simulink library "controller_lib"  (R2022b)
settings: Solver=VariableStepAuto  StartTime=0.0  StopTime=10.0  RelTol=1e-3
libraries: battery_monitor_lib x1, driver_interface_lib x1, governor_lib x1, motor_interface_lib x1, vehicle_dynamics_lib x1
settings Model: Creator=dr_pa  LastModifiedBy=dr_pa

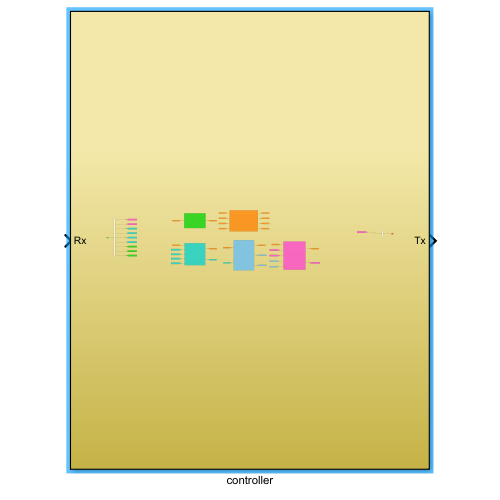
[thumbnail: Simulink's stored preview of the top-level diagram]
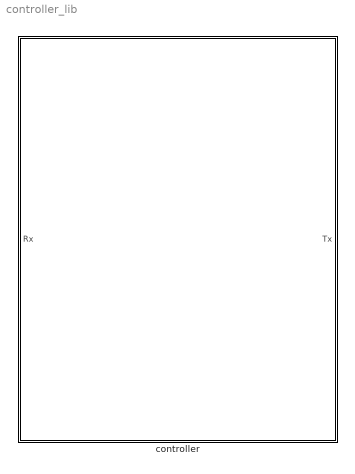
== system controller_lib ==
  controller : Subsystem

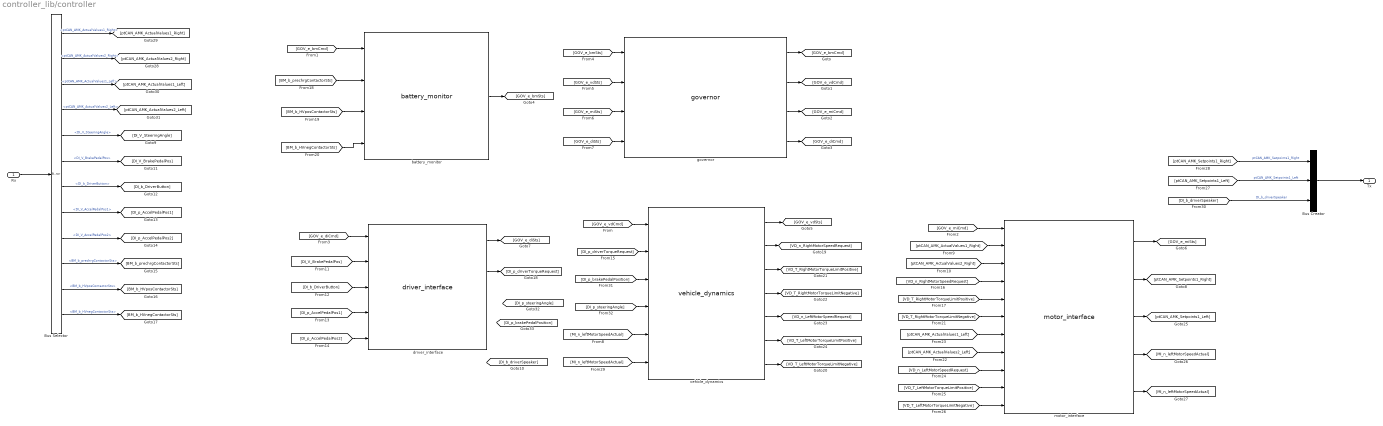
== system controller_lib/controller ==
  Rx : Inport
  Bus Creator : BusCreator  Inputs=3
  Bus Selector : BusSelector  OutputSignals=ptCAN_AMK_ActualValues1_Right,ptCAN_AMK_ActualValues2_Right,ptCAN_AMK_ActualValues1_Left,ptCAN_AMK_ActualValues2_Left,DI_V_SteeringAngle,DI_V_BrakePedalPos,DI_b_DriverButton,DI_V_AccelPedalPos1,DI_V_AccelPedalPos2,BM_b_prechrgContactorSts,BM_b_HVposContactorSts,BM_b_HVnegContactorSts
  battery_monitor : battery_monitor_lib/battery_monitor  SystemSampleTime=-1  VariantActivationTime=update diagram  Latency=0  AutoFrameSizeCalculation=off
  driver_interface : driver_interface_lib/driver_interface  SystemSampleTime=-1  VariantActivationTime=update diagram  Latency=0  AutoFrameSizeCalculation=off
  governor : governor_lib/governor  SystemSampleTime=-1  VariantActivationTime=update diagram  Latency=0  AutoFrameSizeCalculation=off
  motor_interface : motor_interface_lib/motor_interface  SystemSampleTime=-1  VariantActivationTime=update diagram  Latency=0  AutoFrameSizeCalculation=off
  vehicle_dynamics : vehicle_dynamics_lib/vehicle_dynamics  SystemSampleTime=-1  VariantActivationTime=update diagram  Latency=0  AutoFrameSizeCalculation=off
  Tx : Outport
  wires:
  governor/1 -> [GOV_e_bmCmd]
  [GOV_e_vdCmd] -> vehicle_dynamics/1
  governor/2 -> [GOV_e_vdCmd]
  governor/3 -> [GOV_e_miCmd]
  [GOV_e_miCmd] -> motor_interface/1
  governor/4 -> [GOV_e_diCmd]
  [GOV_e_diCmd] -> driver_interface/1
  battery_monitor/1 -> [GOV_e_bmSts]
  [GOV_e_bmSts] -> governor/1
  vehicle_dynamics/1 -> [GOV_e_vdSts]
  [GOV_e_vdSts] -> governor/2
  motor_interface/1 -> [GOV_e_miSts]
  [GOV_e_miSts] -> governor/3
  [GOV_e_diSts] -> governor/4
  driver_interface/1 -> [GOV_e_diSts]
  Bus Creator/1 -> Tx/1
  [ptCAN_AMK_Setpoints1_Right] -> Bus Creator/1  "ptCAN_AMK_Setpoints1_Right"
  motor_interface/2 -> [ptCAN_AMK_Setpoints1_Right]
  [ptCAN_AMK_ActualValues1_Right] -> motor_interface/2
  [ptCAN_AMK_ActualValues2_Right] -> motor_interface/3
  Bus Selector/6 -> [DI_V_BrakePedalPos]  "<DI_V_BrakePedalPos>"
  Bus Selector/7 -> [DI_b_DriverButton]  "<DI_b_DriverButton>"
  Bus Selector/8 -> [DI_p_AccelPedalPos1]  "<DI_V_AccelPedalPos1>"
  Bus Selector/9 -> [DI_p_AccelPedalPos2]  "<DI_V_AccelPedalPos2>"
  Bus Selector/10 -> [BM_b_prechrgContactorSts]  "<BM_b_prechrgContactorSts>"
  Bus Selector/11 -> [BM_b_HVposContactorSts]  "<BM_b_HVposContactorSts>"
  Bus Selector/12 -> [BM_b_HVnegContactorSts]  "<BM_b_HVnegContactorSts>"
  [DI_V_BrakePedalPos] -> driver_interface/2
  [DI_b_DriverButton] -> driver_interface/3
  [DI_p_AccelPedalPos1] -> driver_interface/4
  [DI_p_AccelPedalPos2] -> driver_interface/5
  driver_interface/2 -> [DI_p_driverTorqueRequest]
  vehicle_dynamics/2 -> [VD_n_RightMotorSpeedRequest]
  vehicle_dynamics/3 -> [VD_T_RightMotorTorqueLimitPositive]
  [DI_p_driverTorqueRequest] -> vehicle_dynamics/2
  [VD_n_RightMotorSpeedRequest] -> motor_interface/4
  [VD_T_RightMotorTorqueLimitPositive] -> motor_interface/5
  [BM_b_prechrgContactorSts] -> battery_monitor/2
  [BM_b_HVposContactorSts] -> battery_monitor/3
  [BM_b_HVnegContactorSts] -> battery_monitor/4
  [GOV_e_bmCmd] -> battery_monitor/1
  vehicle_dynamics/4 -> [VD_T_RightMotorTorqueLimitNegative]
  vehicle_dynamics/5 -> [VD_n_LeftMotorSpeedRequest]
  vehicle_dynamics/7 -> [VD_T_LeftMotorTorqueLimitNegative]
  vehicle_dynamics/6 -> [VD_T_LeftMotorTorqueLimitPositive]
  [VD_T_RightMotorTorqueLimitNegative] -> motor_interface/6
  [ptCAN_AMK_ActualValues1_Left] -> motor_interface/7
  [VD_n_LeftMotorSpeedRequest] -> motor_interface/9
  [ptCAN_AMK_ActualValues2_Left] -> motor_interface/8
  [VD_T_LeftMotorTorqueLimitPositive] -> motor_interface/10
  [VD_T_LeftMotorTorqueLimitNegative] -> motor_interface/11
  motor_interface/3 -> [ptCAN_AMK_Setpoints1_Left]
  [ptCAN_AMK_Setpoints1_Left] -> Bus Creator/2  "ptCAN_AMK_Setpoints1_Left"
  motor_interface/5 -> [MI_n_leftMotorSpeedActual]
  motor_interface/4 -> [MI_n_leftMotorSpeedActual]
  [MI_n_leftMotorSpeedActual] -> vehicle_dynamics/6
  [MI_n_leftMotorSpeedActual] -> vehicle_dynamics/5
  Bus Selector/1 -> [ptCAN_AMK_ActualValues1_Right]  "<ptCAN_AMK_ActualValues1_Right>"
  Bus Selector/2 -> [ptCAN_AMK_ActualValues2_Right]  "<ptCAN_AMK_ActualValues2_Right>"
  Bus Selector/3 -> [ptCAN_AMK_ActualValues1_Left]  "<ptCAN_AMK_ActualValues1_Left>"
  Bus Selector/4 -> [ptCAN_AMK_ActualValues2_Left]  "<ptCAN_AMK_ActualValues2_Left>"
  Bus Selector/5 -> [DI_V_SteeringAngle]  "<DI_V_SteeringAngle>"
  [DI_b_driverSpeaker] -> Bus Creator/3  "DI_b_driverSpeaker"
  [DI_p_steeringAngle] -> vehicle_dynamics/4
  [DI_p_brakePedalPosition] -> vehicle_dynamics/3
  Rx/1 -> Bus Selector/1
